simulink model "Djaber"  (Simulink 7.3)
settings: Solver=ode45  StartTime=0.0  StopTime=10.0  RelTol=1e-3
settings Model: Creator=Etudiant  LastModifiedBy=Etudiant

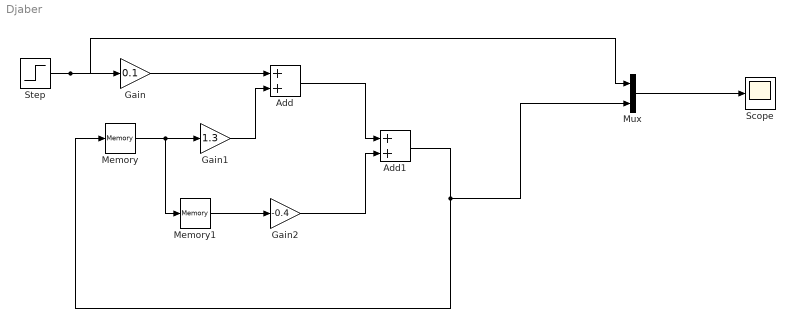
== system Djaber ==
  Add : Sum  OutDataType=fixdt(1, 16)  OutScaling=2^-10
  Add1 : Sum  OutDataType=fixdt(1, 16)  OutScaling=2^-10
  Gain : Gain  Gain=0.1  ParameterDataType=fixdt(1, 16)  ParameterScaling=2^0  OutDataType=fixdt(1, 16)  OutScaling=2^0
  Gain1 : Gain  Gain=1.3  ParameterDataType=fixdt(1, 16)  ParameterScaling=2^0  OutDataType=fixdt(1, 16)  OutScaling=2^0
  Gain2 : Gain  Gain=-0.4  ParameterDataType=fixdt(1, 16)  ParameterScaling=2^0  OutDataType=fixdt(1, 16)  OutScaling=2^0
  Memory : Memory
  Memory1 : Memory
  Mux : Mux  Inputs=2
  Scope : Scope
  Step : Step  SampleTime=0.1
  wires:
  Step/1 -> Gain/1, Mux/1
  Gain/1 -> Add/1
  Memory/1 -> Gain1/1, Memory1/1
  Gain1/1 -> Add/2
  Memory1/1 -> Gain2/1
  Gain2/1 -> Add1/2
  Add/1 -> Add1/1
  Add1/1 -> Memory/1, Mux/2
  Mux/1 -> Scope/1
